simulink model "OpenLoopNonLinearModelActuatorLag"  (R2016a)
settings: Solver=ode1  StartTime=0  StopTime=30  FixedStep=0.05  MaxStep=1e-3  MinStep=1e-5  RelTol=1e-3
values from neighbouring files (symbols this model uses):
  K_AMP = 3    [setup_lab_heli_3d.m]
  par = [Kf;mh;mw;mf;mb;Lh;La;Lw;g;F_v1;F_c1;ta]    [setup_lab_heli_3d.m]
  VMAX_AMP = 24    [setup_lab_heli_3d.m]
  VMAX_DAC = 10    [setup_lab_heli_3d.m]
  X0 = [elev_0;0;0;0;0;0;0;0]    [setup_lab_heli_3d.m]
libraries: simulink_extras x1
settings Model: Creator=ap4614  LastModifiedBy=jcg216
settings SolverCC: InitialStep=1e-3
settings DataIOCC: SaveFormat=Array
settings HardwareCC: ProdBitPerPointer=32  ProdLargestAtomicFloat=None  ProdIntDivRoundTo=Undefined  ProdEndianess=Unspecified  ProdWordSize=32  ProdHWDeviceType=32-bit Generic
settings ModelReferenceCC: PropagateSignalLabelsOutOfModel=off
settings ConfigComp: CovModelRefEnable=Off

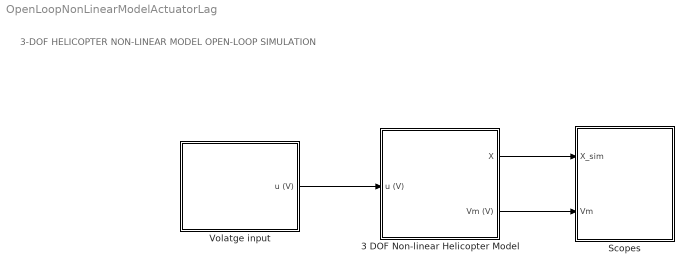
== system OpenLoopNonLinearModelActuatorLag ==
  note: 3-DOF HELICOPTER NON-LINEAR MODEL
      | OPEN-LOOP SIMULATION
  3 DOF Non-linear Helicopter Model : Subsystem
  Scopes : Subsystem
  Volatge input : Subsystem
  wires:
  3 DOF Non-linear Helicopter Model/1("X ") -> Scopes/1(X_sim)
  3 DOF Non-linear Helicopter Model/2(Vm (V)) -> Scopes/2(Vm)
  Volatge input/1(u (V)) -> 3 DOF Non-linear Helicopter Model/1(u (V))

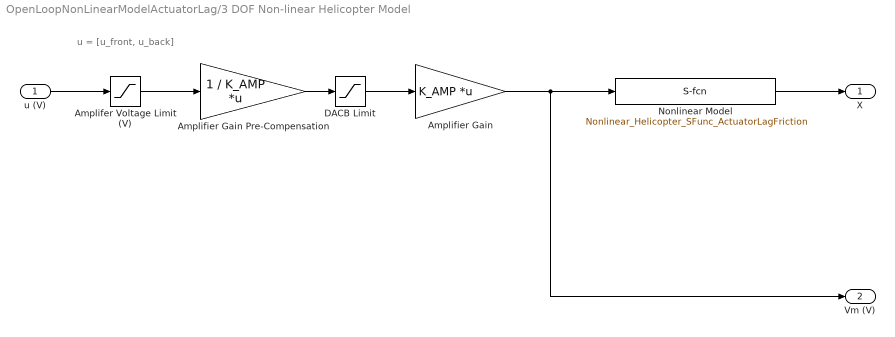
== system OpenLoopNonLinearModelActuatorLag/3 DOF Non-linear Helicopter Model ==
  note: u = [u_front, u_back]
  u (V) : Inport
  " Nonlinear Model" : S-Function  FunctionName=Nonlinear_Helicopter_SFunc_ActuatorLagFriction  Parameters=par,X0  SFunctionDeploymentMode=off  EnableBusSupport=off
  Amplifer Voltage Limit (V) : Saturate  UpperLimit=VMAX_AMP  LowerLimit=-VMAX_AMP
  Amplifier Gain : Gain  Gain=K_AMP  Multiplication=Matrix(K*u)  SaturateOnIntegerOverflow=on  OutDataTypeStr=Inherit: Same as input  ParamDataTypeStr=Inherit: Same as input
  Amplifier Gain Pre-Compensation : Gain  Gain=1 / K_AMP  Multiplication=Matrix(K*u)  SaturateOnIntegerOverflow=on  OutDataTypeStr=Inherit: Same as input  ParamDataTypeStr=Inherit: Same as input
  DACB Limit : Saturate  UpperLimit=VMAX_DAC  LowerLimit=-VMAX_DAC
  "X " : Outport
  Vm (V) : Outport  Port=2
  wires:
  u (V)/1 -> Amplifer Voltage Limit (V)/1
  Amplifer Voltage Limit (V)/1 -> Amplifier Gain Pre-Compensation/1
  Amplifier Gain Pre-Compensation/1 -> DACB Limit/1
  DACB Limit/1 -> Amplifier Gain/1
  Amplifier Gain/1 -> " Nonlinear Model"/1, Vm (V)/1
  " Nonlinear Model"/1 -> "X "/1

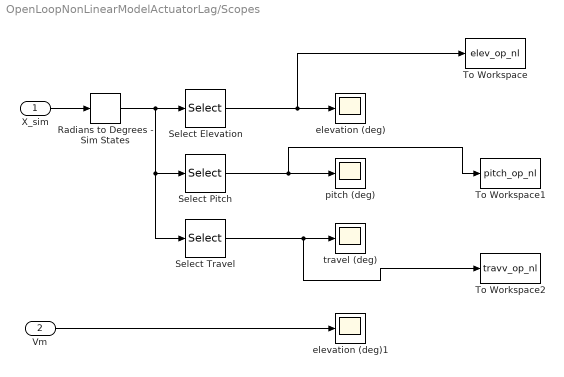
== system OpenLoopNonLinearModelActuatorLag/Scopes ==
  X_sim : Inport
  Vm : Inport  Port=2
  Radians to Degrees - Sim States : simulink_extras/Transformations/Radians to Degrees
  Select Elevation : Selector  InputPortWidth=8  IndexOptions=Index vector (dialog)  Indices=1  OutputSizes=1
  Select Pitch : Selector  InputPortWidth=8  IndexOptions=Index vector (dialog)  Indices=2  OutputSizes=1
  Select Travel : Selector  InputPortWidth=8  IndexOptions=Index vector (dialog)  Indices=3  OutputSizes=1
  To Workspace : ToWorkspace  VariableName=elev_op_nl  SampleTime=-1
  To Workspace1 : ToWorkspace  VariableName=pitch_op_nl  SampleTime=-1
  To Workspace2 : ToWorkspace  VariableName=travv_op_nl  SampleTime=-1
  elevation (deg) : Scope
  elevation (deg)1 : Scope
  pitch (deg) : Scope
  travel (deg) : Scope
  wires:
  Radians to Degrees - Sim States/1 -> Select Elevation/1, Select Pitch/1, Select Travel/1
  X_sim/1 -> Radians to Degrees - Sim States/1
  Vm/1 -> elevation (deg)1/1
  Select Pitch/1 -> To Workspace1/1, pitch (deg)/1
  Select Travel/1 -> To Workspace2/1, travel (deg)/1
  Select Elevation/1 -> To Workspace/1, elevation (deg)/1

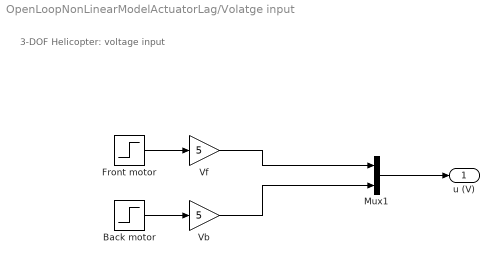
== system OpenLoopNonLinearModelActuatorLag/Volatge input ==
  note: 3-DOF Helicopter: voltage input
  Back motor : Step  SampleTime=0
  Front motor : Step  SampleTime=0
  Mux1 : Mux  Inputs=2
  "Vb " : Gain  Gain=5
  Vf : Gain  Gain=5
  u (V) : Outport
  wires:
  Mux1/1 -> u (V)/1
  Front motor/1 -> Vf/1
  Back motor/1 -> "Vb "/1
  Vf/1 -> Mux1/1
  "Vb "/1 -> Mux1/2
